simulink model "diffusion_hs_sim_sol"  (R2023b)
settings: Solver=ode3  StartTime=0.0  StopTime=100  FixedStep=0.01  RelTol=1e-3
values from neighbouring files (symbols this model uses):
  A = -2*eye(dim)    [diffusion_hs_par_sol.m]    (also in diffusion_par_sol.m)
  B = zeros(dim,1)    [diffusion_hs_par_sol.m]
  C = zeros(1,dim)    [diffusion_hs_par_sol.m]    (also in diffusion_par_sol.m)
  dim = 10    [diffusion_hs_par_sol.m]    (also in diffusion_par_sol.m)
  L_des = acker(A',C',p_obs_des)'    [diffusion_hs_par_sol.m]    (also in diffusion_par_sol.m = acker(A',C',lambda_des)')
settings Model: Creator=jerome  LastModifiedBy=jerome
settings ModelReferenceCC: EnableRefExpFcnMdlSchedulingChecks=on

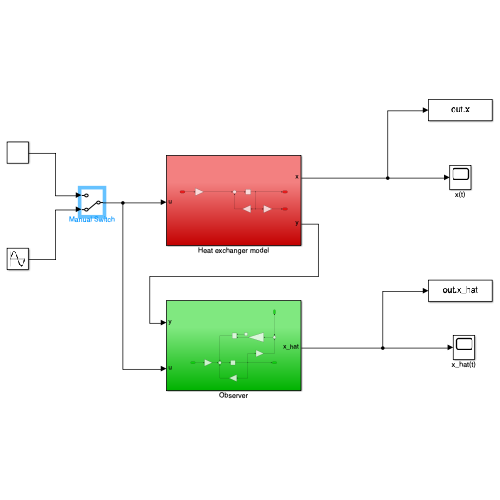
[thumbnail: Simulink's stored preview of the top-level diagram]
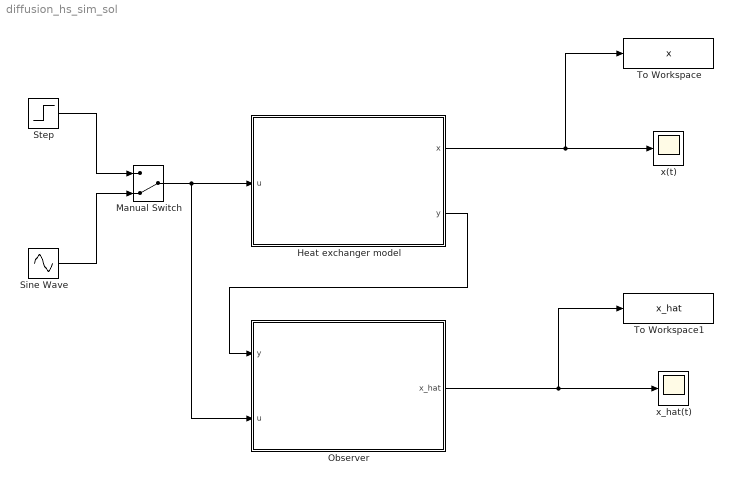
== system diffusion_hs_sim_sol ==
  Heat exchanger model : Subsystem
  Manual Switch : ManualSwitch  CurrentSetting=0
  Observer : Subsystem
  Sine Wave : Sin  Amplitude=6  Bias=3  Frequency=0.5  SampleTime=0
  Step : Step  Time=30  After=10  SampleTime=0
  To Workspace : ToWorkspace  VariableName=x  SampleTime=-1
      settings: Decimation=100
  To Workspace1 : ToWorkspace  VariableName=x_hat  SampleTime=-1
      settings: Decimation=100
  x(t) : Scope
  x_hat(t) : Scope
  wires:
  Heat exchanger model/1(x) -> To Workspace/1, x(t)/1
  Heat exchanger model/2(y) -> Observer/1(y)
  Manual Switch/1 -> Observer/2(u), Heat exchanger model/1(u)
  Observer/1(x_hat) -> To Workspace1/1, x_hat(t)/1
  Step/1 -> Manual Switch/1
  Sine Wave/1 -> Manual Switch/2

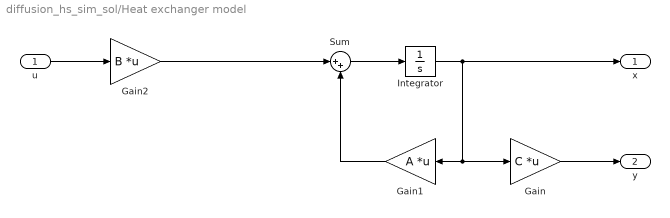
== system diffusion_hs_sim_sol/Heat exchanger model ==
  u : Inport
  Gain : Gain  Gain=C  Multiplication=Matrix(K*u) (u vector)
  Gain1 : Gain  Gain=A  Multiplication=Matrix(K*u) (u vector)
  Gain2 : Gain  Gain=B  Multiplication=Matrix(K*u) (u vector)
  Integrator : Integrator  InitialCondition=randi(20,dim,1)
  Sum : Sum  Inputs=|++
  x : Outport
  y : Outport  Port=2
  wires:
  Integrator/1 -> Gain1/1, Gain/1, x/1
  u/1 -> Gain2/1
  Gain/1 -> y/1
  Sum/1 -> Integrator/1
  Gain1/1 -> Sum/2
  Gain2/1 -> Sum/1

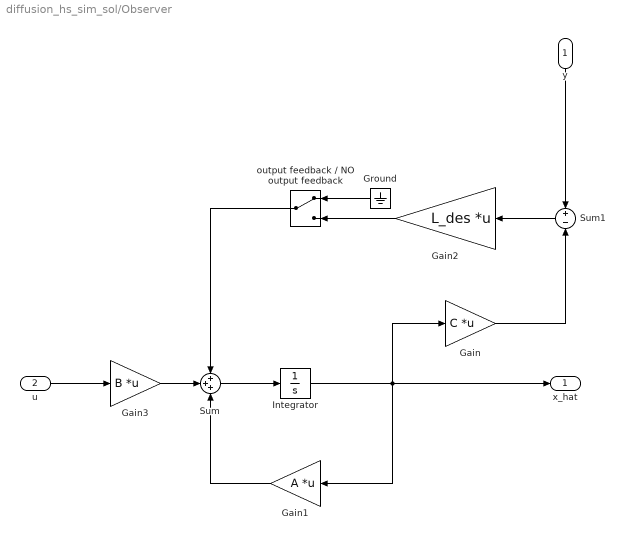
== system diffusion_hs_sim_sol/Observer ==
  y : Inport
  u : Inport  Port=2
  Gain : Gain  Gain=C  Multiplication=Matrix(K*u) (u vector)
  Gain1 : Gain  Gain=A  Multiplication=Matrix(K*u) (u vector)
  Gain2 : Gain  Gain=L_des  Multiplication=Matrix(K*u) (u vector)
  Gain3 : Gain  Gain=B  Multiplication=Matrix(K*u) (u vector)
  Ground : Ground
  Integrator : Integrator  InitialCondition=zeros(dim,1)
  Sum : Sum  Inputs=+++
  Sum1 : Sum  Inputs=+-
  output feedback / NO output feedback : ManualSwitch
  x_hat : Outport
  wires:
  Integrator/1 -> Gain1/1, Gain/1, x_hat/1
  Sum/1 -> Integrator/1
  Gain/1 -> Sum1/2
  y/1 -> Sum1/1
  Sum1/1 -> Gain2/1
  Gain1/1 -> Sum/3
  Gain3/1 -> Sum/2
  u/1 -> Gain3/1
  Gain2/1 -> output feedback / NO output feedback/2
  output feedback / NO output feedback/1 -> Sum/1
  Ground/1 -> output feedback / NO output feedback/1
